simulink model "HighLevelTool"  (R2019b)
settings: Solver=FixedStepDiscrete  StartTime=0.0  StopTime=60.0  FixedStep=0.1  RelTol=1e-3  EnableMultiTasking=on
settings Model: Creator=covasanvictor  LastModifiedBy=covasanvictor
settings SolverCC: AutoInsertRateTranBlk=on
settings OptimizationCC: LifeSpan=inf
settings DebuggingCC: SFUnexpectedBacktrackingDiag=warning  SFNoUnconditionalDefaultTransitionDiag=warning  SFExecutionAtInitializationDiag=none  ArithmeticOperatorsInVariantConditions=warning
settings SFSimCC: SimUseLocalCustomCode=off  CustomCodeUndefinedFunction=UseInterfaceOnly
settings RTWCC: RTWUseLocalCustomCode=off
settings CodeAppCC: StateflowObjectComments=on
settings GRTTargetCC: TargetLangStandard=C89/C90 (ANSI)
settings ConfigComp: CovMetricSettings=dw  CovHtmlReporting=on  CovSaveCumulativeToWorkspaceVar=on  CovSaveSingleToWorkspaceVar=on  CovShowResultsExplorer=off  CovExternalEMLEnable=off

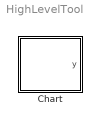
== system HighLevelTool ==
  Chart : Stateflow chart  TreatAsAtomicUnit=on

== stateflow chart HighLevelTool/Chart ==
  note: LEDS FOR: Calibration(flashing red vs steady for), Battery(steady Orange), Pause(Green steady for take a break, flashing for )
  state Standby
    entry: y = -1;
    ButtonState = PollButton();
    RecordErgonomics();
    BatteryStates = CheckBattery();
    RecordTimeSinceLastBreak();
    CheckCalibration();
    ScanForScrewHeads();
    DetectScrewDriver();
    SelectCorrectDriver();
    connection = CheckInternetConn(); % then if ON send data
    CheckEncoder();
    while(~button)
    if(RecordTimeSinceLastBreak()>BreakThreshold)
    {
    Flash(BreakLED,)
    }
    if(connection){
    uploadData();
    clearData();
    }
    }
  state Run % Parent State
    state High % Child State
      ApproachedScrew= a;
      entry: ButtonState = b;
      CalibrationState = c;
      if(ApproachedScrew&&
      ButtonState&&
      CalibrationState){
      ApplyTorque(ScrewType)
      }
      RecordTorque();
      RecordScrewHole();
      if(RecordTorque()~=TorqueScrewType(ScrewType))
      Flash(Decalibrated, ON, secondsWarning)
      if(outsideTorqueRange(ScrewType){
      Flash(calibrationWarning, ON,secondsWarning)
      }
    state Low % Child State
      entry: y = 1;
    (default) -> High % Child State
    High % Child State -> Low % Child State : after(1,sec)
    Low % Child State -> High % Child State : after(1,sec)
  note: In this state machine, s tate Run contains 2 child states High and Low. The state machine switches between High and Low after 1 sec.
  (default) -> Run % Parent State [order 1]
  Run % Parent State -> ? : after(30,sec)
  (default) -> Run % Parent State [order 2] : after(5,sec)
  data: y output
